simulink model "Modulationofsys"  (R2021a)
settings: Solver=VariableStepAuto  StartTime=0.0  StopTime=5  RelTol=1e-3
settings Model: Creator=bahet  LastModifiedBy=Jubin Thomas

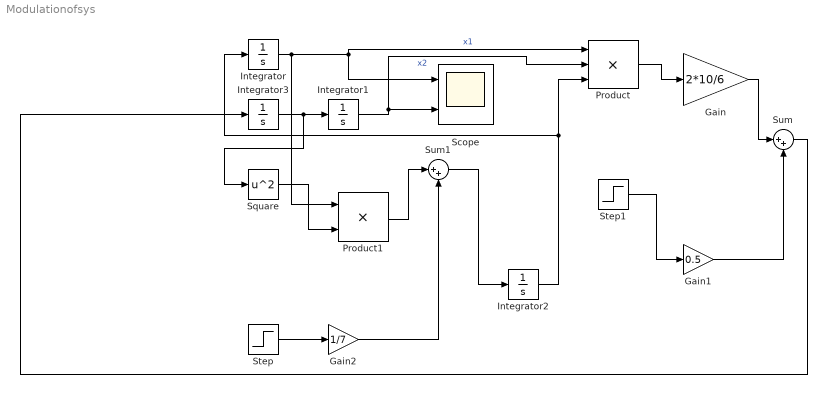
== system Modulationofsys ==
  Gain : Gain  Gain=2*10/6
  Gain1 : Gain  Gain=0.5
  Gain2 : Gain  Gain=1/7
  Integrator : Integrator
  Integrator1 : Integrator
  Integrator2 : Integrator  InitialCondition=0.01
  Integrator3 : Integrator
  Product : Product  Inputs=3
  Product1 : Product
  Scope : Scope  NumInputPorts=2
  Square : Math  Operator=square  SaturateOnIntegerOverflow=on
  Step : Step  Before=1  After=0  SampleTime=0
  Step1 : Step  Before=1  After=0  SampleTime=0
  Sum : Sum  Inputs=|++
  Sum1 : Sum  Inputs=|++
  wires:
  Integrator/1 -> Scope/1, Product/1, Product1/1  "x1"
  Integrator1/1 -> Product/2, Scope/2  "x2"
  Integrator3/1 -> Square/1, Integrator1/1
  Step1/1 -> Gain1/1
  Product1/1 -> Sum1/1
  Integrator2/1 -> Product/3, Integrator/1
  Sum1/1 -> Integrator2/1
  Gain2/1 -> Sum1/2
  Gain1/1 -> Sum/2
  Sum/1 -> Integrator3/1
  Product/1 -> Gain/1
  Step/1 -> Gain2/1
  Gain/1 -> Sum/1
  Square/1 -> Product1/2
